simulink model "APP_ChkSig"  (R2020b)
settings: configuration reference "cs_ert" (kept outside this file)
model workspace (MAT data in the model file):
  APP_ChkSig_DT = 10
values from neighbouring files (symbols this model uses):
  APP_rThresAliveDet_C = 20.0    [APP_ChkSig.sldd]
  APP_swtAliveDetEna_C = 0    [APP_ChkSig.sldd]
  APP_tiAliveDebHiLo_C = 300.0    [APP_ChkSig.sldd]
  APP_tiAliveDebLoHi_C = 0.0    [APP_ChkSig.sldd]
undefined symbols (not defined in the file or in its folder): Switch
libraries: sllib x2, simulink x2
settings Model: DataDictionary=APP_ChkSig.sldd  EnableAccessToBaseWorkspace=off  Creator=zhoutinglin  LastModifiedBy=zhoutinglin
settings ConfigSetRef: SourceName=cs_ert

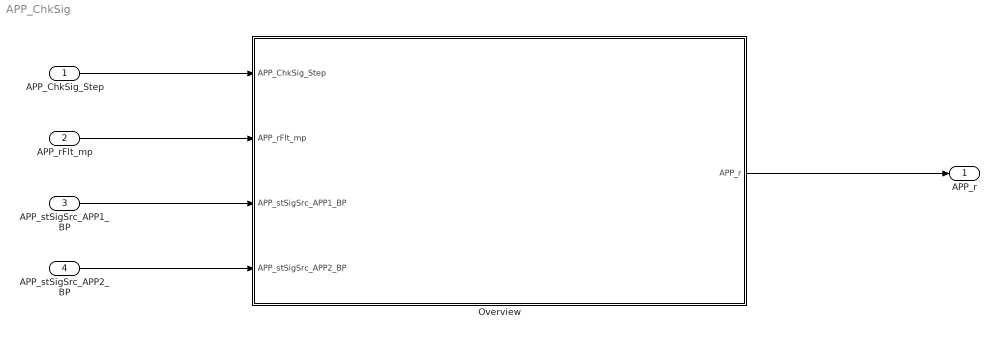
== system APP_ChkSig ==
  APP_ChkSig_Step : Inport  OutputFunctionCall=on
  APP_rFlt_mp : Inport  Description=Acceleration pedal position filtered value  Port=2  OutMin=0  OutMax=100  OutDataTypeStr=Percent  Unit=%  PortDimensions=[1 1]
  APP_stSigSrc_APP1_BP : Inport  Description=Sensor 1 is the reference variable, Sensor 2 value is defective  Port=3  OutMin=0  OutMax=1  OutDataTypeStr=boolean  PortDimensions=[1 1]
  APP_stSigSrc_APP2_BP : Inport  Description=Sensor 2 is the reference variable,Sensor1 value is defective  Port=4  OutMin=0  OutMax=1  OutDataTypeStr=boolean  PortDimensions=[1 1]
  Overview : Subsystem
  APP_r : Outport  Description=Acceleration pedal sensor 1 value after fault handling  OutMin=0  OutMax=100  OutDataTypeStr=Percent  Unit=%  PortDimensions=[1 1]  VectorParamsAs1DForOutWhenUnconnected=off
  wires:
  APP_ChkSig_Step/1 -> Overview/1(APP_ChkSig_Step)
  APP_rFlt_mp/1 -> Overview/2(APP_rFlt_mp)
  APP_stSigSrc_APP1_BP/1 -> Overview/3(APP_stSigSrc_APP1_BP)
  APP_stSigSrc_APP2_BP/1 -> Overview/4(APP_stSigSrc_APP2_BP)
  Overview/1(APP_r) -> APP_r/1

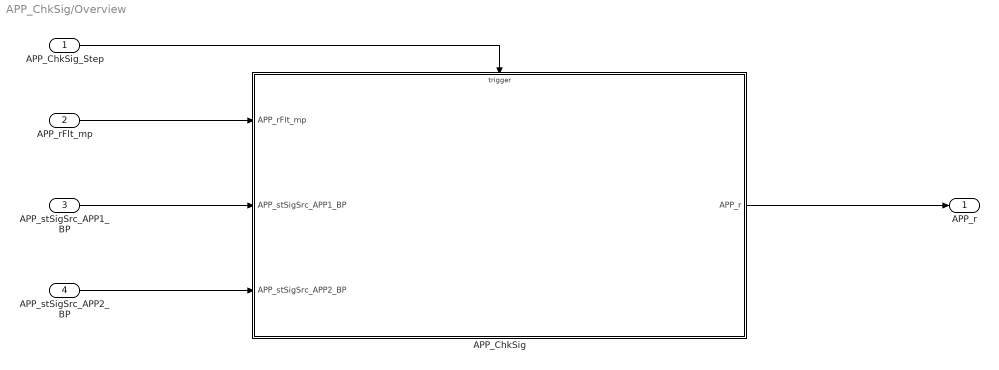
== system APP_ChkSig/Overview ==
  APP_ChkSig_Step : Inport
  APP_rFlt_mp : Inport  Port=2
  APP_stSigSrc_APP1_BP : Inport  Port=3
  APP_stSigSrc_APP2_BP : Inport  Port=4
  APP_ChkSig : Subsystem
  APP_r : Outport  VectorParamsAs1DForOutWhenUnconnected=off
  wires:
  APP_rFlt_mp/1 -> APP_ChkSig/1(APP_rFlt_mp)
  APP_stSigSrc_APP1_BP/1 -> APP_ChkSig/2(APP_stSigSrc_APP1_BP)
  APP_stSigSrc_APP2_BP/1 -> APP_ChkSig/3(APP_stSigSrc_APP2_BP)
  APP_ChkSig/1(APP_r) -> APP_r/1
  APP_ChkSig_Step/1 -> APP_ChkSig/Trigger

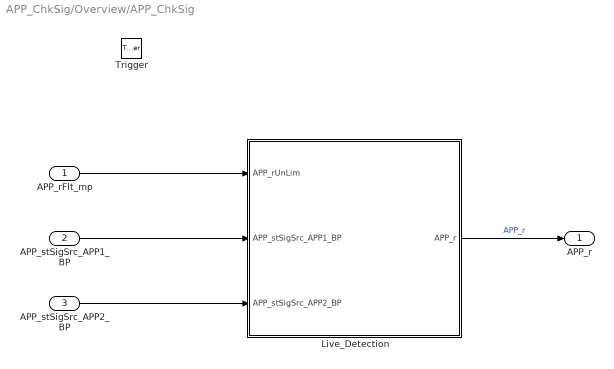
== system APP_ChkSig/Overview/APP_ChkSig ==
  APP_rFlt_mp : Inport  Tag=%
  APP_stSigSrc_APP1_BP : Inport  Port=2
  APP_stSigSrc_APP2_BP : Inport  Port=3
  Trigger : TriggerPort  TriggerType=function-call  VariantControl=Variant  PortDimensions=1
  Live_Detection : Subsystem
  APP_r : Outport  Tag=%  VectorParamsAs1DForOutWhenUnconnected=off
  wires:
  Live_Detection/1(APP_r) -> APP_r/1  "APP_r"
  APP_rFlt_mp/1 -> Live_Detection/1(APP_rUnLim)
  APP_stSigSrc_APP2_BP/1 -> Live_Detection/3(APP_stSigSrc_APP2_BP)
  APP_stSigSrc_APP1_BP/1 -> Live_Detection/2(APP_stSigSrc_APP1_BP)

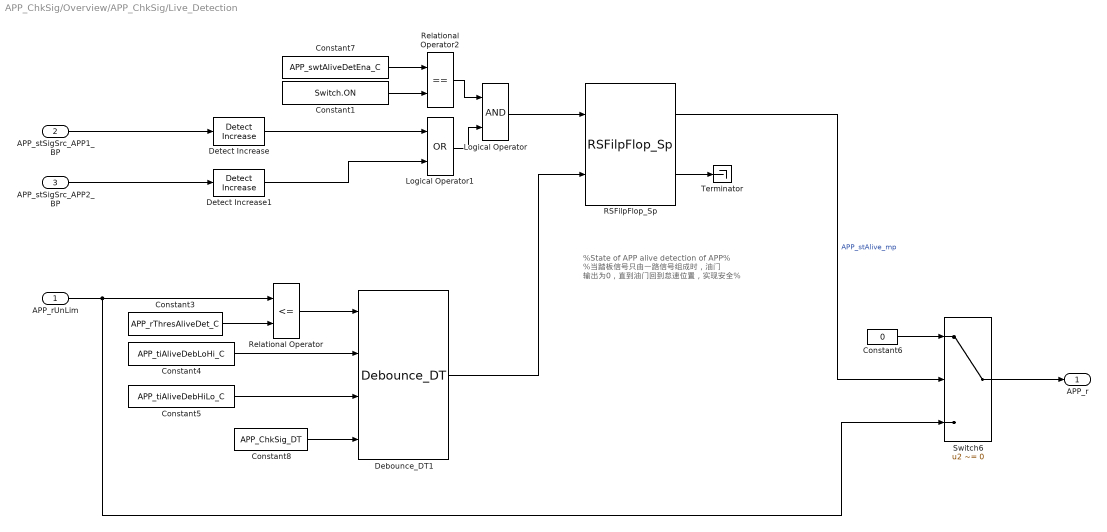
== system APP_ChkSig/Overview/APP_ChkSig/Live_Detection ==
  note: %State of APP alive detection of APP%
      | %当踏板信号只由一路信号组成时，油门
      | 输出为0，直到油门回到怠速位置，实现安全%
  APP_rUnLim : Inport
  APP_stSigSrc_APP1_BP : Inport  Port=2
  APP_stSigSrc_APP2_BP : Inport  Port=3
  Constant1 : Constant  Value=Switch.ON  OutDataTypeStr=Inherit: Inherit via back propagation
  Constant3 : Constant  Value=APP_rThresAliveDet_C
  Constant4 : Constant  Value=APP_tiAliveDebLoHi_C
  Constant5 : Constant  Value=APP_tiAliveDebHiLo_C
  Constant6 : Constant  Value=0  OutDataTypeStr=Inherit: Inherit via back propagation
  Constant7 : Constant  Value=APP_swtAliveDetEna_C
  Constant8 : Constant  Value=APP_ChkSig_DT  OutDataTypeStr=Inherit: Inherit via back propagation
  Debounce_DT1 : sllib/Timer and counter operators/Debounce_DT
      settings: SourceProductName=sllib
  Detect Increase : simulink/Logic and Bit Operations/Detect Increase  vinit=0.0  OutDataTypeStr=boolean
  Detect Increase1 : simulink/Logic and Bit Operations/Detect Increase  vinit=0.0  OutDataTypeStr=boolean
  Logical Operator : Logic  OutDataTypeStr=boolean
  Logical Operator1 : Logic  Operator=OR  OutDataTypeStr=boolean
  RSFilpFlop_Sp : sllib/Logical symbols/RSFilpFlop_Sp  InitialCondition=0
      settings: AttributesFormatString=State Initial=%<InitialCondition>  SourceProductName=sllib
  Relational Operator : RelationalOperator  Operator=<=  OutDataTypeStr=boolean  RndMeth=Nearest  InputSameDT=on
  Relational Operator2 : RelationalOperator  Operator===  OutDataTypeStr=boolean  RndMeth=Nearest  InputSameDT=on
  Switch6 : Switch  Criteria=u2 ~= 0  InputSameDT=on
  Terminator : Terminator
  APP_r : Outport  VectorParamsAs1DForOutWhenUnconnected=off
  wires:
  Logical Operator/1 -> RSFilpFlop_Sp/1
  RSFilpFlop_Sp/2 -> Terminator/1
  Logical Operator1/1 -> Logical Operator/2
  Relational Operator/1 -> Debounce_DT1/1
  APP_stSigSrc_APP1_BP/1 -> Detect Increase/1
  Debounce_DT1/1 -> RSFilpFlop_Sp/2
  Constant1/1 -> Relational Operator2/2
  Constant7/1 -> Relational Operator2/1
  Relational Operator2/1 -> Logical Operator/1
  RSFilpFlop_Sp/1 -> Switch6/2  "APP_stAlive_mp"
  Constant5/1 -> Debounce_DT1/3
  Constant4/1 -> Debounce_DT1/2
  Constant3/1 -> Relational Operator/2
  Constant8/1 -> Debounce_DT1/4
  APP_rUnLim/1 -> Switch6/3, Relational Operator/1
  Constant6/1 -> Switch6/1
  Detect Increase/1 -> Logical Operator1/1
  APP_stSigSrc_APP2_BP/1 -> Detect Increase1/1
  Detect Increase1/1 -> Logical Operator1/2
  Switch6/1 -> APP_r/1
